simulink model "nl_obsv_hydrotrans_dspace"  (R2021b)
settings: Solver=ode1be  StartTime=0.0  StopTime=inf  FixedStep=ts  MaxStep=ts
PostLoadFcn:
  | if any(exist('dsrtsu_mdlpostloadfcn', 'file') ~= 0), dsrtsu_mdlpostloadfcn('Execute', bdroot); end
InitFcn:
  | , if any(exist('rtifpga_mdlclblib', 'file') ~= 0), rtifpga_mdlclblib('Init', bdroot); end,
  | , if any(exist('dsmpb_private', 'file') ~= 0), dsmpb_private('dsmpb_mdlclblib', 'Init', bdroot); end,
values from neighbouring files (symbols this model uses):
  bd = 5e-2    (= 0.05)    [init_nlobsv_hd.m]
  bf = 0.1    [init_nlobsv_hd.m]
  bm = 0.02    [init_nlobsv_hd.m]
  bp = 0.02    [init_nlobsv_hd.m]
  bulk = 8.36e9    (= 8360000000)    [init_nlobsv_hd.m]
  engine_speed_ref_rpm = 1940    [init_nlobsv_hd.m]
  Jm = 0.05    [init_nlobsv_hd.m]
  Jp = 0.05    [init_nlobsv_hd.m]
  kdrag = 0.01    [init_nlobsv_hd.m]
  kdrag_model = 0.01    [init_nlobsv_hd.m]
  ki_engine = 2.5e-1    (= 0.25)    [init_nlobsv_hd.m]
  kleak = 1e-6    (= 1e-06)    [init_nlobsv_hd.m]
  kp_engine = 2.5e-2    (= 0.025)    [init_nlobsv_hd.m]
  max_domega_m_dt = omega_m_nom_rpm/4    (= 1000)    [init_nlobsv_hd.m]
  ntg = 1    [init_nlobsv_hd.m]
  omega_m_nom_rpm = 4000    [init_nlobsv_hd.m]
  omega_m_ref = 3200    [init_nlobsv_hd.m]
  P0 = eye(4)    [init_nlobsv_hd.m]
  q11 = 10    [init_nlobsv_hd.m]
  q22 = 10    [init_nlobsv_hd.m]
  q33 = 10    [init_nlobsv_hd.m]
  q44 = 2e3    (= 2000)    [init_nlobsv_hd.m]
  ts = 1e-3    (= 0.001)    [init_nlobsv_hd.m]
  tstep = 20    [init_nlobsv_hd.m]
  Vm_nom = 280    [init_nlobsv_hd.m]
  Vp_nom = 210    [init_nlobsv_hd.m]
undefined symbols (not defined in the file or in its folder): consumption, DiscIntNeverNeededParam, rpm_base, rpm_consumption, torque_base, torque_consumption, torque_friction_base
libraries: fl_lib x70, nesl_utility x36, linear_swashplate_ctrl_lib x4, variable_displacement_motor_2_lib x2, variable_displacement_pump_2_lib x2, fixed_displacement_pump_lib x2, relief_valve_lib x2, inverse_shuttle_valve_lib x2, engine_speed_ctrl_kinputs_lib x1, ice_lib x1, gear2_lib x1, flexshaft_lib x1
(part 2 of 2)

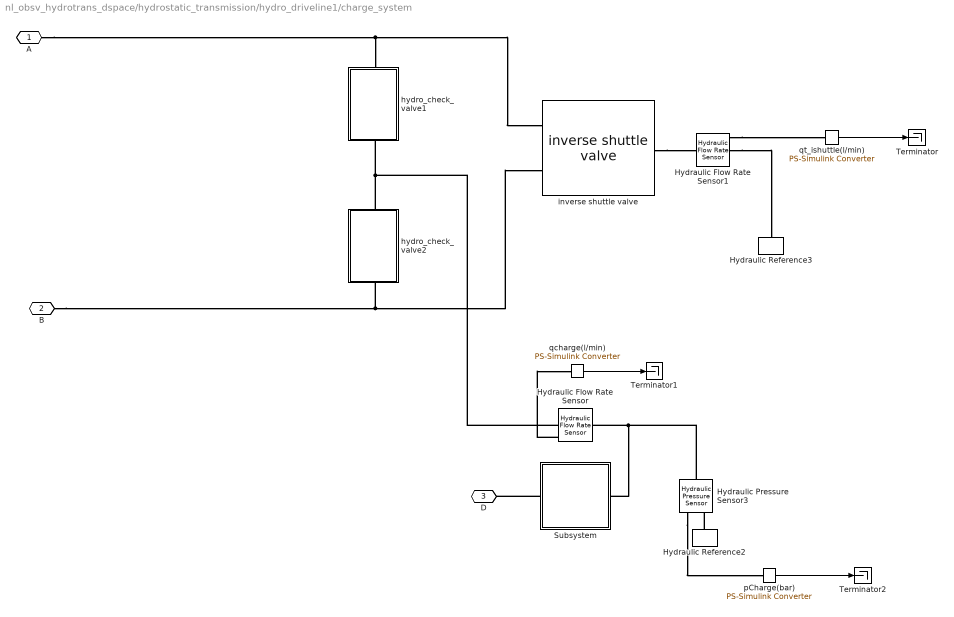
== system nl_obsv_hydrotrans_dspace/hydrostatic_transmission/hydro_driveline1/charge_system ==
  Hydraulic Flow Rate Sensor : fl_lib/Hydraulic/Hydraulic Sensors/Hydraulic Flow Rate Sensor
  Hydraulic Flow Rate Sensor1 : fl_lib/Hydraulic/Hydraulic Sensors/Hydraulic Flow Rate Sensor
  Hydraulic Pressure Sensor3 : fl_lib/Hydraulic/Hydraulic Sensors/Hydraulic Pressure Sensor
  Hydraulic Reference2 : fl_lib/Hydraulic/Hydraulic Elements/Hydraulic Reference
  Hydraulic Reference3 : fl_lib/Hydraulic/Hydraulic Elements/Hydraulic Reference
  Subsystem : Subsystem
  Terminator : Terminator
  Terminator1 : Terminator
  Terminator2 : Terminator
  hydro_check_valve1 : Subsystem
      settings: PortSchema="{\"entries\":[{\"content\":{\"sides\":[{\"content\":{\"connectorIds\":[]},\"type\":\"ConnectorPlacement.EquallySpacedRectSide\",\"uuid\":\"a69fbb91-2279-4dfd-af6f-16497d5f1538\"},{\"content\":{\"connectorIds\":[],\"side\":\"RIGHT\"},\"type\":\"ConnectorPlacement.EquallySpacedRectSide\",\"uuid\":\"52e95d44-b7af-4ccc-8556-a2abd2e724e0\"},{\"content\":{\"connectorIds\":[\"LConn1\"],\"side\":\"TOP\"},\"type\":\"ConnectorPlacement.EquallySpacedRectSide\",\"uuid\":\"2d8c071e-4cd0-4b83-8d45-c175cb858754\"},{\"content\":{\"connectorIds\":[\"RConn1\"],\"side\":\"BOTTOM\"},\"type\":\"ConnectorPlacement.EquallySpacedRectSide\",\"uuid\":\"1baec9dc-757c-4f21-904a-6fc08de72ce1\"}]},\"type\":\"ConnectorPlacement.EquallySpacedConnector\",\"uuid\":\"76990e53-6cb0-4bfe-8c9e-427c41b785f2\"}],\"packageUris\":[\"http://schema.mathworks.com/mf0/Connector/19700101\"],\"version\":\"1.0\"}"
  hydro_check_valve2 : Subsystem
      settings: PortSchema="{\"entries\":[{\"content\":{\"sides\":[{\"content\":{\"connectorIds\":[]},\"type\":\"ConnectorPlacement.EquallySpacedRectSide\",\"uuid\":\"a69fbb91-2279-4dfd-af6f-16497d5f1538\"},{\"content\":{\"connectorIds\":[],\"side\":\"RIGHT\"},\"type\":\"ConnectorPlacement.EquallySpacedRectSide\",\"uuid\":\"52e95d44-b7af-4ccc-8556-a2abd2e724e0\"},{\"content\":{\"connectorIds\":[\"LConn1\"],\"side\":\"TOP\"},\"type\":\"ConnectorPlacement.EquallySpacedRectSide\",\"uuid\":\"2d8c071e-4cd0-4b83-8d45-c175cb858754\"},{\"content\":{\"connectorIds\":[\"RConn1\"],\"side\":\"BOTTOM\"},\"type\":\"ConnectorPlacement.EquallySpacedRectSide\",\"uuid\":\"1baec9dc-757c-4f21-904a-6fc08de72ce1\"}]},\"type\":\"ConnectorPlacement.EquallySpacedConnector\",\"uuid\":\"76990e53-6cb0-4bfe-8c9e-427c41b785f2\"}],\"packageUris\":[\"http://schema.mathworks.com/mf0/Connector/19700101\"],\"version\":\"1.0\"}"
  inverse shuttle valve : inverse_shuttle_valve_lib/inverse shuttle valve  pnom=32 bar  dp_crack=0 bar  dp_reg=0 bar  x_rv_max=2 mm  a0=(2*pi*10)^2 1/s^2  a1=2*2*pi*10 1/s  leak=5e-12 m^3/s/Pa  qA_specify=off  qA_priority=None  qA=0 m^3/s  qA_nominal_specify=off  qA_nominal_unit=m^3/s  qA_nominal_value=1  qB_specify=off  qB_priority=None  qB=0 m^3/s  qB_nominal_specify=off  qB_nominal_unit=m^3/s  qB_nominal_value=1  qP_specify=off  qP_priority=None  qP=0 m^3/s  qP_nominal_specify=off  qP_nominal_unit=m^3/s  qP_nominal_value=1  dp_specify=off  dp_priority=None  dp=0 Pa  dp_nominal_specify=off  dp_nominal_unit=Pa  dp_nominal_value=1  dpAP_specify=off  dpAP_priority=None  dpAP=0 Pa  dpAP_nominal_specify=off  dpAP_nominal_unit=Pa  dpAP_nominal_value=1  dpBP_specify=off  dpBP_priority=None  dpBP=0 Pa  dpBP_nominal_specify=off  dpBP_nominal_unit=Pa  dpBP_nominal_value=1  x_rv_AP_specify=off  x_rv_AP_priority=None  x_rv_AP=0 m  x_rv_AP_nominal_specify=off  x_rv_AP_nominal_unit=m  x_rv_AP_nominal_value=1  x_rv_BP_specify=off  x_rv_BP_priority=None  x_rv_BP=0 m  x_rv_BP_nominal_specify=off  x_rv_BP_nominal_unit=m  x_rv_BP_nominal_value=1  x_rv_AP_flt_specify=off  x_rv_AP_flt_priority=None  x_rv_AP_flt=0 m  x_rv_AP_flt_nominal_specify=off  x_rv_AP_flt_nominal_unit=m  x_rv_AP_flt_nominal_value=1  x_rv_BP_flt_specify=off  x_rv_BP_flt_priority=None  x_rv_BP_flt=0 m  x_rv_BP_flt_nominal_specify=off  x_rv_BP_flt_nominal_unit=m  x_rv_BP_flt_nominal_value=1
      settings: InternalSimscapePortConfiguration="{\"Bottom\":[],\"Left\":[{\"id\":\"cA\",\"label\":\"cA\",\"type\":\"foundation.hydraulic.hydraulic\"},{\"id\":\"cB\",\"label\":\"cB\",\"type\":\"foundation.hydraulic.hydraulic\"}],\"Right\":[{\"id\":\"cP\",\"label\":\"cP\",\"type\":\"foundation.hydraulic.hydraulic\"}],\"Top\":[]}"
  pCharge(bar) : nesl_utility/PS-Simulink Converter  PhysicalDomain=network_engine_domain  SubClassName=ps_output  LeftPortType=input  RightPortType=output  PseudoPeriodic=off  Frequencies=[]  Unit=bar  AffineConversion=on
      settings: SourceProductBaseCode=PW,SS
  qcharge(l/min) : nesl_utility/PS-Simulink Converter  PhysicalDomain=network_engine_domain  SubClassName=ps_output  LeftPortType=input  RightPortType=output  PseudoPeriodic=off  Frequencies=[]  Unit=l/min  AffineConversion=on
      settings: SourceProductBaseCode=PW,SS
  qt_ishuttle(l/min) : nesl_utility/PS-Simulink Converter  PhysicalDomain=network_engine_domain  SubClassName=ps_output  LeftPortType=input  RightPortType=output  PseudoPeriodic=off  Frequencies=[]  Unit=l/min  AffineConversion=on
      settings: SourceProductBaseCode=PW,SS
  A : PMIOPort  Side=Left
  B : PMIOPort  Port=2  Side=Right
  D : PMIOPort  Port=3  Side=Right
  wires:
  qt_ishuttle(l/min)/1 -> Terminator/1
  qcharge(l/min)/1 -> Terminator1/1
  pCharge(bar)/1 -> Terminator2/1
  connections:
  hydro_check_valve2/LConn1 -- Hydraulic Flow Rate Sensor/RConn2 -- hydro_check_valve1/LConn1
  A/RConn1 -- inverse shuttle valve/LConn1 -- hydro_check_valve1/RConn1
  B/RConn1 -- inverse shuttle valve/LConn2 -- hydro_check_valve2/RConn1
  Hydraulic Flow Rate Sensor/RConn1 -- qcharge(l/min)/LConn1
  Hydraulic Pressure Sensor3/LConn1 -- Subsystem/RConn1 -- Hydraulic Flow Rate Sensor/LConn1
  Subsystem/LConn1 -- D/RConn1
  Hydraulic Pressure Sensor3/RConn2 -- pCharge(bar)/LConn1
  Hydraulic Reference2/LConn1 -- Hydraulic Pressure Sensor3/RConn1
  Hydraulic Flow Rate Sensor1/RConn2 -- Hydraulic Reference3/LConn1
  Hydraulic Flow Rate Sensor1/RConn1 -- qt_ishuttle(l/min)/LConn1
  inverse shuttle valve/RConn1 -- Hydraulic Flow Rate Sensor1/LConn1

== system nl_obsv_hydrotrans_dspace/hydrostatic_transmission/hydro_driveline1/vd_ctrl_motor ==
  vd_ref : Inport
  Linear swashplate ctrl2 : linear_swashplate_ctrl_lib/Linear swashplate ctrl  a12=1 1/s  b2=1 1/m/s  k1=100 m  k2=20.5 m  N=5 m  kv=20  xv_specify=off  xv_priority=None  xv=0 m  xv_nominal_specify=off  xv_nominal_unit=m  xv_nominal_value=1  D1_specify=off  D1_priority=None  D1=0  D1_nominal_specify=off  D1_nominal_unit=1  D1_nominal_value=1  D2_specify=off  D2_priority=None  D2=0  D2_nominal_specify=off  D2_nominal_unit=1  D2_nominal_value=1
      settings: InternalSimscapePortConfiguration="{\"Bottom\":[],\"Left\":[{\"id\":\"D_ref\",\"label\":\"Dref\",\"type\":\"input\"}],\"Right\":[{\"id\":\"Dout\",\"label\":\"Dout\",\"type\":\"output\"}],\"Top\":[]}"
  Simulink-PS Converter3 : nesl_utility/Simulink-PS Converter  PhysicalDomain=network_engine_domain  SubClassName=ps_input  LeftPortType=input  RightPortType=output  PseudoPeriodic=off  Frequencies=[]  NoiseDistribution=none  NoiseParameters=[]  Unit=1  AffineConversion=off  FilteringAndDerivatives=provide  SimscapeFilterOrder=1  InputFilterTimeConstant=0.001  UdotUserProvided=0
      settings: SourceProductBaseCode=PW,SS
  vd : PMIOPort  Side=Right
  wires:
  vd_ref/1 -> Simulink-PS Converter3/1
  connections:
  Simulink-PS Converter3/RConn1 -- Linear swashplate ctrl2/LConn1
  Linear swashplate ctrl2/RConn1 -- vd/RConn1

== system nl_obsv_hydrotrans_dspace/hydrostatic_transmission/hydro_driveline1/vd_ctrl_pump ==
  vd_ref : Inport
  Linear swashplate ctrl2 : linear_swashplate_ctrl_lib/Linear swashplate ctrl  a12=1 1/s  b2=1 1/m/s  k1=100 m  k2=20.5 m  N=5 m  kv=20  xv_specify=off  xv_priority=None  xv=0 m  xv_nominal_specify=off  xv_nominal_unit=m  xv_nominal_value=1  D1_specify=off  D1_priority=None  D1=0  D1_nominal_specify=off  D1_nominal_unit=1  D1_nominal_value=1  D2_specify=off  D2_priority=None  D2=0  D2_nominal_specify=off  D2_nominal_unit=1  D2_nominal_value=1
      settings: InternalSimscapePortConfiguration="{\"Bottom\":[],\"Left\":[{\"id\":\"D_ref\",\"label\":\"Dref\",\"type\":\"input\"}],\"Right\":[{\"id\":\"Dout\",\"label\":\"Dout\",\"type\":\"output\"}],\"Top\":[]}"
  Simulink-PS Converter3 : nesl_utility/Simulink-PS Converter  PhysicalDomain=network_engine_domain  SubClassName=ps_input  LeftPortType=input  RightPortType=output  PseudoPeriodic=off  Frequencies=[]  NoiseDistribution=none  NoiseParameters=[]  Unit=1  AffineConversion=off  FilteringAndDerivatives=provide  SimscapeFilterOrder=1  InputFilterTimeConstant=0.001  UdotUserProvided=0
      settings: SourceProductBaseCode=PW,SS
  vd : PMIOPort  Side=Right
  wires:
  vd_ref/1 -> Simulink-PS Converter3/1
  connections:
  Simulink-PS Converter3/RConn1 -- Linear swashplate ctrl2/LConn1
  Linear swashplate ctrl2/RConn1 -- vd/RConn1

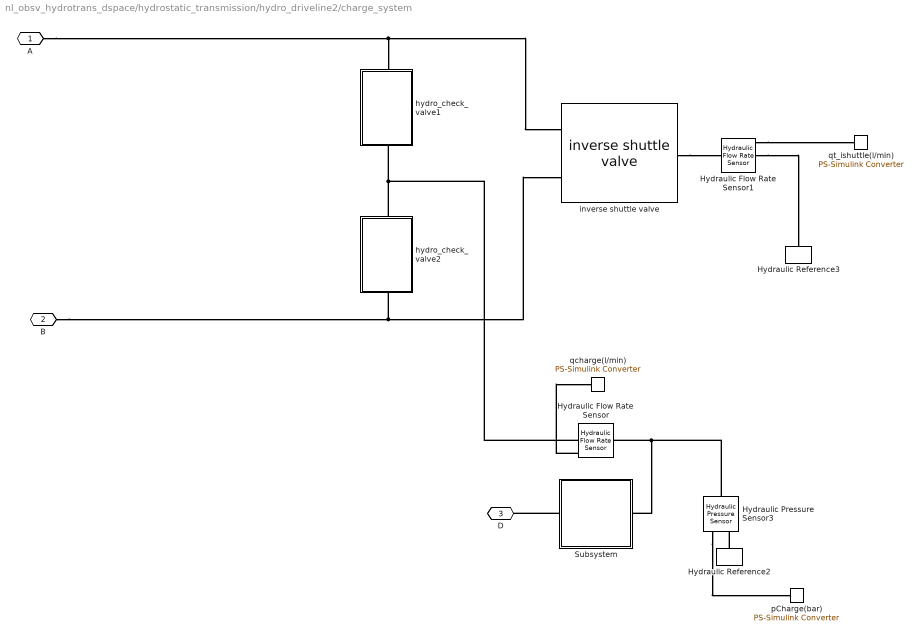
== system nl_obsv_hydrotrans_dspace/hydrostatic_transmission/hydro_driveline2/charge_system ==
  Hydraulic Flow Rate Sensor : fl_lib/Hydraulic/Hydraulic Sensors/Hydraulic Flow Rate Sensor
  Hydraulic Flow Rate Sensor1 : fl_lib/Hydraulic/Hydraulic Sensors/Hydraulic Flow Rate Sensor
  Hydraulic Pressure Sensor3 : fl_lib/Hydraulic/Hydraulic Sensors/Hydraulic Pressure Sensor
  Hydraulic Reference2 : fl_lib/Hydraulic/Hydraulic Elements/Hydraulic Reference
  Hydraulic Reference3 : fl_lib/Hydraulic/Hydraulic Elements/Hydraulic Reference
  Subsystem : Subsystem
  hydro_check_valve1 : Subsystem
      settings: PortSchema="{\"entries\":[{\"content\":{\"sides\":[{\"content\":{\"connectorIds\":[]},\"type\":\"ConnectorPlacement.EquallySpacedRectSide\",\"uuid\":\"a69fbb91-2279-4dfd-af6f-16497d5f1538\"},{\"content\":{\"connectorIds\":[],\"side\":\"RIGHT\"},\"type\":\"ConnectorPlacement.EquallySpacedRectSide\",\"uuid\":\"52e95d44-b7af-4ccc-8556-a2abd2e724e0\"},{\"content\":{\"connectorIds\":[\"LConn1\"],\"side\":\"TOP\"},\"type\":\"ConnectorPlacement.EquallySpacedRectSide\",\"uuid\":\"2d8c071e-4cd0-4b83-8d45-c175cb858754\"},{\"content\":{\"connectorIds\":[\"RConn1\"],\"side\":\"BOTTOM\"},\"type\":\"ConnectorPlacement.EquallySpacedRectSide\",\"uuid\":\"1baec9dc-757c-4f21-904a-6fc08de72ce1\"}]},\"type\":\"ConnectorPlacement.EquallySpacedConnector\",\"uuid\":\"76990e53-6cb0-4bfe-8c9e-427c41b785f2\"}],\"packageUris\":[\"http://schema.mathworks.com/mf0/Connector/19700101\"],\"version\":\"1.0\"}"
  hydro_check_valve2 : Subsystem
      settings: PortSchema="{\"entries\":[{\"content\":{\"sides\":[{\"content\":{\"connectorIds\":[]},\"type\":\"ConnectorPlacement.EquallySpacedRectSide\",\"uuid\":\"a69fbb91-2279-4dfd-af6f-16497d5f1538\"},{\"content\":{\"connectorIds\":[],\"side\":\"RIGHT\"},\"type\":\"ConnectorPlacement.EquallySpacedRectSide\",\"uuid\":\"52e95d44-b7af-4ccc-8556-a2abd2e724e0\"},{\"content\":{\"connectorIds\":[\"LConn1\"],\"side\":\"TOP\"},\"type\":\"ConnectorPlacement.EquallySpacedRectSide\",\"uuid\":\"2d8c071e-4cd0-4b83-8d45-c175cb858754\"},{\"content\":{\"connectorIds\":[\"RConn1\"],\"side\":\"BOTTOM\"},\"type\":\"ConnectorPlacement.EquallySpacedRectSide\",\"uuid\":\"1baec9dc-757c-4f21-904a-6fc08de72ce1\"}]},\"type\":\"ConnectorPlacement.EquallySpacedConnector\",\"uuid\":\"76990e53-6cb0-4bfe-8c9e-427c41b785f2\"}],\"packageUris\":[\"http://schema.mathworks.com/mf0/Connector/19700101\"],\"version\":\"1.0\"}"
  inverse shuttle valve : inverse_shuttle_valve_lib/inverse shuttle valve  pnom=32 bar  dp_crack=0 bar  dp_reg=0 bar  x_rv_max=2 mm  a0=(2*pi*10)^2 1/s^2  a1=2*2*pi*10 1/s  leak=5e-12 m^3/s/Pa  qA_specify=off  qA_priority=None  qA=0 m^3/s  qA_nominal_specify=off  qA_nominal_unit=m^3/s  qA_nominal_value=1  qB_specify=off  qB_priority=None  qB=0 m^3/s  qB_nominal_specify=off  qB_nominal_unit=m^3/s  qB_nominal_value=1  qP_specify=off  qP_priority=None  qP=0 m^3/s  qP_nominal_specify=off  qP_nominal_unit=m^3/s  qP_nominal_value=1  dp_specify=off  dp_priority=None  dp=0 Pa  dp_nominal_specify=off  dp_nominal_unit=Pa  dp_nominal_value=1  dpAP_specify=off  dpAP_priority=None  dpAP=0 Pa  dpAP_nominal_specify=off  dpAP_nominal_unit=Pa  dpAP_nominal_value=1  dpBP_specify=off  dpBP_priority=None  dpBP=0 Pa  dpBP_nominal_specify=off  dpBP_nominal_unit=Pa  dpBP_nominal_value=1  x_rv_AP_specify=off  x_rv_AP_priority=None  x_rv_AP=0 m  x_rv_AP_nominal_specify=off  x_rv_AP_nominal_unit=m  x_rv_AP_nominal_value=1  x_rv_BP_specify=off  x_rv_BP_priority=None  x_rv_BP=0 m  x_rv_BP_nominal_specify=off  x_rv_BP_nominal_unit=m  x_rv_BP_nominal_value=1  x_rv_AP_flt_specify=off  x_rv_AP_flt_priority=None  x_rv_AP_flt=0 m  x_rv_AP_flt_nominal_specify=off  x_rv_AP_flt_nominal_unit=m  x_rv_AP_flt_nominal_value=1  x_rv_BP_flt_specify=off  x_rv_BP_flt_priority=None  x_rv_BP_flt=0 m  x_rv_BP_flt_nominal_specify=off  x_rv_BP_flt_nominal_unit=m  x_rv_BP_flt_nominal_value=1
      settings: InternalSimscapePortConfiguration="{\"Bottom\":[],\"Left\":[{\"id\":\"cA\",\"label\":\"cA\",\"type\":\"foundation.hydraulic.hydraulic\"},{\"id\":\"cB\",\"label\":\"cB\",\"type\":\"foundation.hydraulic.hydraulic\"}],\"Right\":[{\"id\":\"cP\",\"label\":\"cP\",\"type\":\"foundation.hydraulic.hydraulic\"}],\"Top\":[]}"
  pCharge(bar) : nesl_utility/PS-Simulink Converter  PhysicalDomain=network_engine_domain  SubClassName=ps_output  LeftPortType=input  RightPortType=output  PseudoPeriodic=off  Frequencies=[]  Unit=bar  AffineConversion=on
      settings: SourceProductBaseCode=PW,SS
  qcharge(l/min) : nesl_utility/PS-Simulink Converter  PhysicalDomain=network_engine_domain  SubClassName=ps_output  LeftPortType=input  RightPortType=output  PseudoPeriodic=off  Frequencies=[]  Unit=l/min  AffineConversion=on
      settings: SourceProductBaseCode=PW,SS
  qt_ishuttle(l/min) : nesl_utility/PS-Simulink Converter  PhysicalDomain=network_engine_domain  SubClassName=ps_output  LeftPortType=input  RightPortType=output  PseudoPeriodic=off  Frequencies=[]  Unit=l/min  AffineConversion=on
      settings: SourceProductBaseCode=PW,SS
  A : PMIOPort  Side=Left
  B : PMIOPort  Port=2  Side=Right
  D : PMIOPort  Port=3  Side=Right
  connections:
  hydro_check_valve2/LConn1 -- Hydraulic Flow Rate Sensor/RConn2 -- hydro_check_valve1/LConn1
  A/RConn1 -- inverse shuttle valve/LConn1 -- hydro_check_valve1/RConn1
  B/RConn1 -- inverse shuttle valve/LConn2 -- hydro_check_valve2/RConn1
  Hydraulic Flow Rate Sensor/RConn1 -- qcharge(l/min)/LConn1
  Hydraulic Pressure Sensor3/LConn1 -- Subsystem/RConn1 -- Hydraulic Flow Rate Sensor/LConn1
  Subsystem/LConn1 -- D/RConn1
  Hydraulic Pressure Sensor3/RConn2 -- pCharge(bar)/LConn1
  Hydraulic Reference2/LConn1 -- Hydraulic Pressure Sensor3/RConn1
  Hydraulic Flow Rate Sensor1/RConn2 -- Hydraulic Reference3/LConn1
  Hydraulic Flow Rate Sensor1/RConn1 -- qt_ishuttle(l/min)/LConn1
  inverse shuttle valve/RConn1 -- Hydraulic Flow Rate Sensor1/LConn1

== system nl_obsv_hydrotrans_dspace/hydrostatic_transmission/hydro_driveline2/vd_ctrl_motor ==
  vd_ref : Inport
  Linear swashplate ctrl2 : linear_swashplate_ctrl_lib/Linear swashplate ctrl  a12=1 1/s  b2=1 1/m/s  k1=100 m  k2=20.5 m  N=5 m  kv=20  xv_specify=off  xv_priority=None  xv=0 m  xv_nominal_specify=off  xv_nominal_unit=m  xv_nominal_value=1  D1_specify=off  D1_priority=None  D1=0  D1_nominal_specify=off  D1_nominal_unit=1  D1_nominal_value=1  D2_specify=off  D2_priority=None  D2=0  D2_nominal_specify=off  D2_nominal_unit=1  D2_nominal_value=1
      settings: InternalSimscapePortConfiguration="{\"Bottom\":[],\"Left\":[{\"id\":\"D_ref\",\"label\":\"Dref\",\"type\":\"input\"}],\"Right\":[{\"id\":\"Dout\",\"label\":\"Dout\",\"type\":\"output\"}],\"Top\":[]}"
  Simulink-PS Converter3 : nesl_utility/Simulink-PS Converter  PhysicalDomain=network_engine_domain  SubClassName=ps_input  LeftPortType=input  RightPortType=output  PseudoPeriodic=off  Frequencies=[]  NoiseDistribution=none  NoiseParameters=[]  Unit=1  AffineConversion=off  FilteringAndDerivatives=provide  SimscapeFilterOrder=1  InputFilterTimeConstant=0.001  UdotUserProvided=0
      settings: SourceProductBaseCode=PW,SS
  vd : PMIOPort  Side=Right
  wires:
  vd_ref/1 -> Simulink-PS Converter3/1
  connections:
  Linear swashplate ctrl2/RConn1 -- vd/RConn1
  Simulink-PS Converter3/RConn1 -- Linear swashplate ctrl2/LConn1

== system nl_obsv_hydrotrans_dspace/hydrostatic_transmission/hydro_driveline2/vd_ctrl_pump ==
  vd_ref : Inport
  Linear swashplate ctrl2 : linear_swashplate_ctrl_lib/Linear swashplate ctrl  a12=1 1/s  b2=1 1/m/s  k1=100 m  k2=20.5 m  N=5 m  kv=20  xv_specify=off  xv_priority=None  xv=0 m  xv_nominal_specify=off  xv_nominal_unit=m  xv_nominal_value=1  D1_specify=off  D1_priority=None  D1=0  D1_nominal_specify=off  D1_nominal_unit=1  D1_nominal_value=1  D2_specify=off  D2_priority=None  D2=0  D2_nominal_specify=off  D2_nominal_unit=1  D2_nominal_value=1
      settings: InternalSimscapePortConfiguration="{\"Bottom\":[],\"Left\":[{\"id\":\"D_ref\",\"label\":\"Dref\",\"type\":\"input\"}],\"Right\":[{\"id\":\"Dout\",\"label\":\"Dout\",\"type\":\"output\"}],\"Top\":[]}"
  Simulink-PS Converter3 : nesl_utility/Simulink-PS Converter  PhysicalDomain=network_engine_domain  SubClassName=ps_input  LeftPortType=input  RightPortType=output  PseudoPeriodic=off  Frequencies=[]  NoiseDistribution=none  NoiseParameters=[]  Unit=1  AffineConversion=off  FilteringAndDerivatives=provide  SimscapeFilterOrder=1  InputFilterTimeConstant=0.001  UdotUserProvided=0
      settings: SourceProductBaseCode=PW,SS
  vd : PMIOPort  Side=Right
  wires:
  vd_ref/1 -> Simulink-PS Converter3/1
  connections:
  Linear swashplate ctrl2/RConn1 -- vd/RConn1
  Simulink-PS Converter3/RConn1 -- Linear swashplate ctrl2/LConn1

== system nl_obsv_hydrotrans_dspace/hydrostatic_transmission/hydro_driveline1/charge_system/Subsystem ==
  Fixed displacement pump : fixed_displacement_pump_lib/Fixed displacement pump  max_Dv=27 cm^3/rev  inertia_pump=0.05 kg*m^2  oil_vol=2.0 l  bp=0.0025 N*m/(rad/s)  lk=1e-6 m  t_specify=off  t_priority=None  t=0 N*m  t_nominal_specify=off  t_nominal_unit=N*m  t_nominal_value=1  q_specify=off  q_priority=None  q=0 m^3/s  q_nominal_specify=off  q_nominal_unit=m^3/s  q_nominal_value=1  qt_specify=off  qt_priority=None  qt=0 m^3/s  qt_nominal_specify=off  qt_nominal_unit=m^3/s  qt_nominal_value=1  qleak_specify=off  qleak_priority=None  qleak=0 m^3/s  qleak_nominal_specify=off  qleak_nominal_unit=m^3/s  qleak_nominal_value=1  Dv_specify=off  Dv_priority=None  Dv=0 cm^3  Dv_nominal_specify=off  Dv_nominal_unit=cm^3  Dv_nominal_value=1  dp_specify=off  dp_priority=None  dp=0 Pa  dp_nominal_specify=off  dp_nominal_unit=Pa  dp_nominal_value=1  we_specify=off  we_priority=None  we=0 rad/s  we_nominal_specify=off  we_nominal_unit=rad/s  we_nominal_value=1
      settings: InternalSimscapePortConfiguration="{\"Bottom\":[],\"Left\":[{\"id\":\"C\",\"label\":\"C\",\"type\":\"foundation.mechanical.rotational.rotational\"}],\"Right\":[{\"id\":\"A\",\"label\":\"A\",\"type\":\"foundation.hydraulic.hydraulic\"},{\"id\":\"B\",\"label\":\"B\",\"type\":\"foundation.hydraulic.hydraulic\"}],\"Top\":[]}"
  Hydraulic Reference3 : fl_lib/Hydraulic/Hydraulic Elements/Hydraulic Reference
  Hydraulic Reference4 : fl_lib/Hydraulic/Hydraulic Elements/Hydraulic Reference
  relief valve : relief_valve_lib/relief valve  dp_ref=32 bar  pnom=32 bar  p_set=32 bar  p_reg=12 bar  x_rv_max=12.0 mm  qA_specify=off  qA_priority=None  qA=0 m^3/s  qA_nominal_specify=off  qA_nominal_unit=m^3/s  qA_nominal_value=1  qB_specify=off  qB_priority=None  qB=0 m^3/s  qB_nominal_specify=off  qB_nominal_unit=m^3/s  qB_nominal_value=1  dp_specify=off  dp_priority=None  dp=0 Pa  dp_nominal_specify=off  dp_nominal_unit=Pa  dp_nominal_value=1  x_rv_specify=off  x_rv_priority=None  x_rv=0 m  x_rv_nominal_specify=off  x_rv_nominal_unit=m  x_rv_nominal_value=1  x_rv_flt_specify=off  x_rv_flt_priority=None  x_rv_flt=0 m  x_rv_flt_nominal_specify=off  x_rv_flt_nominal_unit=m  x_rv_flt_nominal_value=1
      settings: LogSimulationData=on  InternalSimscapePortConfiguration="{\"Bottom\":[],\"Left\":[{\"id\":\"cA\",\"label\":\"cA\",\"type\":\"foundation.hydraulic.hydraulic\"}],\"Right\":[{\"id\":\"cB\",\"label\":\"cB\",\"type\":\"foundation.hydraulic.hydraulic\"}],\"Top\":[]}"
  ps : PMIOPort  Side=Right
  D : PMIOPort  Port=2  Side=Left
  connections:
  Fixed displacement pump/RConn1 -- ps/RConn1 -- relief valve/LConn1
  Hydraulic Reference4/LConn1 -- relief valve/RConn1
  Fixed displacement pump/RConn2 -- Hydraulic Reference3/LConn1
  Fixed displacement pump/LConn1 -- D/RConn1

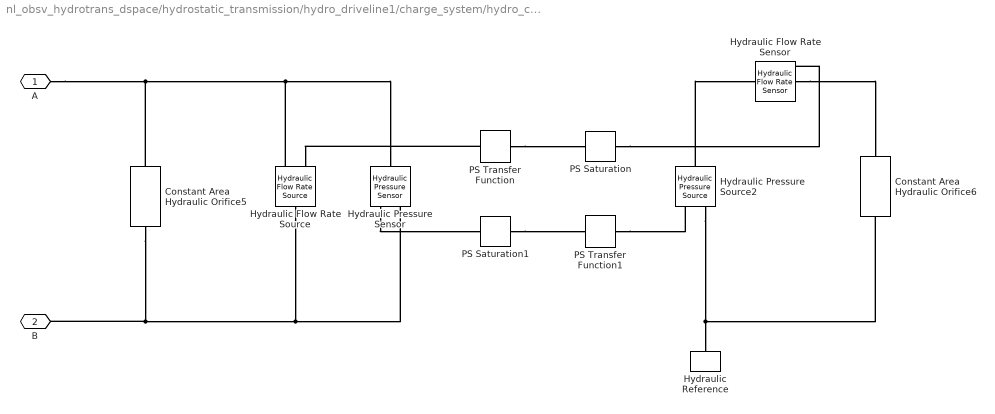
== system nl_obsv_hydrotrans_dspace/hydrostatic_transmission/hydro_driveline1/charge_system/hydro_check_valve1 ==
  Constant Area Hydraulic Orifice5 : fl_lib/Hydraulic/Hydraulic Elements/Constant Area Hydraulic Orifice  area=1e-4 mm^2  C_d=1  lam_spec=1  B_lam=0.999  Re_cr=12  q_specify=off  q_priority=None  q=0.001 m^3/s  q_nominal_specify=off  q_nominal_unit=m^3/s  q_nominal_value=1  p_specify=off  p_priority=None  p=0 Pa  p_nominal_specify=off  p_nominal_unit=Pa  p_nominal_value=1
      settings: SourceProductBaseCode=SS  InternalSimscapePortConfiguration="{\"Bottom\":[],\"Left\":[{\"id\":\"A\",\"label\":\"A\",\"type\":\"foundation.hydraulic.hydraulic\"}],\"Right\":[{\"id\":\"B\",\"label\":\"B\",\"type\":\"foundation.hydraulic.hydraulic\"}],\"Top\":[]}"
  Constant Area Hydraulic Orifice6 : fl_lib/Hydraulic/Hydraulic Elements/Constant Area Hydraulic Orifice  area=4 mm^2  C_d=1  lam_spec=1  B_lam=0.999  Re_cr=12  q_specify=off  q_priority=None  q=0.001 m^3/s  q_nominal_specify=off  q_nominal_unit=m^3/s  q_nominal_value=1  p_specify=off  p_priority=None  p=0 Pa  p_nominal_specify=off  p_nominal_unit=Pa  p_nominal_value=1
      settings: SourceProductBaseCode=SS  InternalSimscapePortConfiguration="{\"Bottom\":[],\"Left\":[{\"id\":\"A\",\"label\":\"A\",\"type\":\"foundation.hydraulic.hydraulic\"}],\"Right\":[{\"id\":\"B\",\"label\":\"B\",\"type\":\"foundation.hydraulic.hydraulic\"}],\"Top\":[]}"
  Hydraulic Flow Rate Sensor : fl_lib/Hydraulic/Hydraulic Sensors/Hydraulic Flow Rate Sensor
  Hydraulic Flow Rate Source : fl_lib/Hydraulic/Hydraulic Sources/Hydraulic Flow Rate Source
      settings: SourceProductBaseCode=SS  InternalSimscapePortConfiguration="{\"Bottom\":[],\"Left\":[{\"id\":\"P\",\"label\":\"P\",\"type\":\"foundation.hydraulic.hydraulic\"}],\"Right\":[{\"id\":\"S\",\"label\":\"S\",\"type\":\"input\"},{\"id\":\"T\",\"label\":\"T\",\"type\":\"foundation.hydraulic.hydraulic\"}],\"Top\":[]}"
  Hydraulic Pressure Sensor : fl_lib/Hydraulic/Hydraulic Sensors/Hydraulic Pressure Sensor
  Hydraulic Pressure Source2 : fl_lib/Hydraulic/Hydraulic Sources/Hydraulic Pressure Source
      settings: SourceProductBaseCode=SS  InternalSimscapePortConfiguration="{\"Bottom\":[],\"Left\":[{\"id\":\"P\",\"label\":\"P\",\"type\":\"foundation.hydraulic.hydraulic\"}],\"Right\":[{\"id\":\"S\",\"label\":\"S\",\"type\":\"input\"},{\"id\":\"T\",\"label\":\"T\",\"type\":\"foundation.hydraulic.hydraulic\"}],\"Top\":[]}"
  Hydraulic Reference : fl_lib/Hydraulic/Hydraulic Elements/Hydraulic Reference
  PS Saturation : fl_lib/Physical Signals/Nonlinear Operators/PS Saturation  upper_limit=inf m^3/s  lower_limit=0 m^3/s
      settings: SourceProductBaseCode=SS
  PS Saturation1 : fl_lib/Physical Signals/Nonlinear Operators/PS Saturation  upper_limit=inf Pa  lower_limit=0 Pa
      settings: SourceProductBaseCode=SS
  PS Transfer Function : fl_lib/Physical Signals/Linear Operators/PS Transfer Function  transfer_function_type=foundation.enum.transfer_function_type.lag  T=ts s  T1=2 s  T2=1 s  y0=0 m^3/s
      settings: SourceProductBaseCode=SS  InternalSimscapePortConfiguration="{\"Bottom\":[],\"Left\":[{\"id\":\"U\",\"label\":\"\",\"type\":\"input\"}],\"Right\":[{\"id\":\"Y\",\"label\":\"\",\"type\":\"output\"}],\"Top\":[]}"
  PS Transfer Function1 : fl_lib/Physical Signals/Linear Operators/PS Transfer Function  transfer_function_type=foundation.enum.transfer_function_type.lag  T=ts s  T1=2 s  T2=1 s  y0=0 Pa
      settings: SourceProductBaseCode=SS  InternalSimscapePortConfiguration="{\"Bottom\":[],\"Left\":[{\"id\":\"U\",\"label\":\"\",\"type\":\"input\"}],\"Right\":[{\"id\":\"Y\",\"label\":\"\",\"type\":\"output\"}],\"Top\":[]}"
  A : PMIOPort  Side=Left
  B : PMIOPort  Port=2  Side=Right
  connections:
  Hydraulic Flow Rate Sensor/RConn2 -- Constant Area Hydraulic Orifice6/LConn1
  Constant Area Hydraulic Orifice6/RConn1 -- Hydraulic Reference/LConn1 -- Hydraulic Pressure Source2/RConn2
  Hydraulic Pressure Source2/LConn1 -- Hydraulic Flow Rate Sensor/LConn1
  Hydraulic Flow Rate Source/LConn1 -- Hydraulic Pressure Sensor/RConn1 -- Constant Area Hydraulic Orifice5/RConn1 -- B/RConn1
  PS Saturation/LConn1 -- Hydraulic Flow Rate Sensor/RConn1
  PS Transfer Function1/RConn1 -- Hydraulic Pressure Source2/RConn1
  Hydraulic Pressure Sensor/RConn2 -- PS Saturation1/LConn1
  Hydraulic Flow Rate Source/RConn2 -- Hydraulic Pressure Sensor/LConn1 -- A/RConn1 -- Constant Area Hydraulic Orifice5/LConn1
  PS Transfer Function/RConn1 -- Hydraulic Flow Rate Source/RConn1
  PS Saturation1/RConn1 -- PS Transfer Function1/LConn1
  PS Transfer Function/LConn1 -- PS Saturation/RConn1

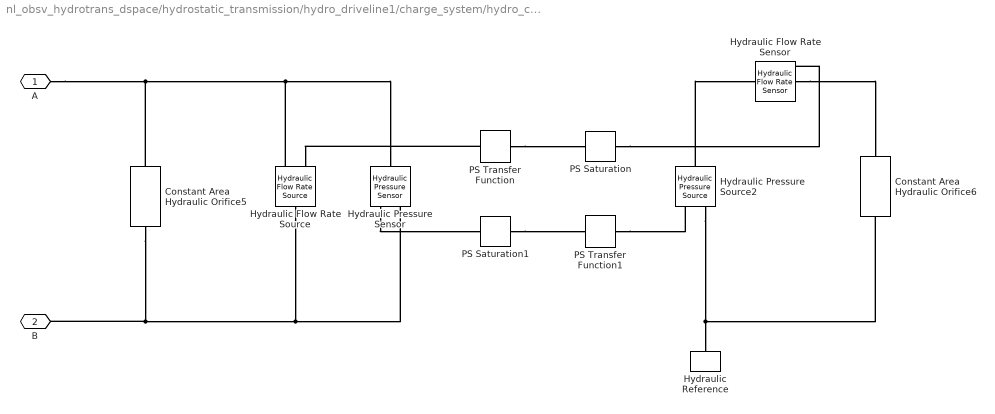
== system nl_obsv_hydrotrans_dspace/hydrostatic_transmission/hydro_driveline1/charge_system/hydro_check_valve2 ==
  Constant Area Hydraulic Orifice5 : fl_lib/Hydraulic/Hydraulic Elements/Constant Area Hydraulic Orifice  area=1e-4 mm^2  C_d=1  lam_spec=1  B_lam=0.999  Re_cr=12  q_specify=off  q_priority=None  q=0.001 m^3/s  q_nominal_specify=off  q_nominal_unit=m^3/s  q_nominal_value=1  p_specify=off  p_priority=None  p=0 Pa  p_nominal_specify=off  p_nominal_unit=Pa  p_nominal_value=1
      settings: SourceProductBaseCode=SS  InternalSimscapePortConfiguration="{\"Bottom\":[],\"Left\":[{\"id\":\"A\",\"label\":\"A\",\"type\":\"foundation.hydraulic.hydraulic\"}],\"Right\":[{\"id\":\"B\",\"label\":\"B\",\"type\":\"foundation.hydraulic.hydraulic\"}],\"Top\":[]}"
  Constant Area Hydraulic Orifice6 : fl_lib/Hydraulic/Hydraulic Elements/Constant Area Hydraulic Orifice  area=4 mm^2  C_d=1  lam_spec=1  B_lam=0.999  Re_cr=12  q_specify=off  q_priority=None  q=0.001 m^3/s  q_nominal_specify=off  q_nominal_unit=m^3/s  q_nominal_value=1  p_specify=off  p_priority=None  p=0 Pa  p_nominal_specify=off  p_nominal_unit=Pa  p_nominal_value=1
      settings: SourceProductBaseCode=SS  InternalSimscapePortConfiguration="{\"Bottom\":[],\"Left\":[{\"id\":\"A\",\"label\":\"A\",\"type\":\"foundation.hydraulic.hydraulic\"}],\"Right\":[{\"id\":\"B\",\"label\":\"B\",\"type\":\"foundation.hydraulic.hydraulic\"}],\"Top\":[]}"
  Hydraulic Flow Rate Sensor : fl_lib/Hydraulic/Hydraulic Sensors/Hydraulic Flow Rate Sensor
  Hydraulic Flow Rate Source : fl_lib/Hydraulic/Hydraulic Sources/Hydraulic Flow Rate Source
      settings: SourceProductBaseCode=SS  InternalSimscapePortConfiguration="{\"Bottom\":[],\"Left\":[{\"id\":\"P\",\"label\":\"P\",\"type\":\"foundation.hydraulic.hydraulic\"}],\"Right\":[{\"id\":\"S\",\"label\":\"S\",\"type\":\"input\"},{\"id\":\"T\",\"label\":\"T\",\"type\":\"foundation.hydraulic.hydraulic\"}],\"Top\":[]}"
  Hydraulic Pressure Sensor : fl_lib/Hydraulic/Hydraulic Sensors/Hydraulic Pressure Sensor
  Hydraulic Pressure Source2 : fl_lib/Hydraulic/Hydraulic Sources/Hydraulic Pressure Source
      settings: SourceProductBaseCode=SS  InternalSimscapePortConfiguration="{\"Bottom\":[],\"Left\":[{\"id\":\"P\",\"label\":\"P\",\"type\":\"foundation.hydraulic.hydraulic\"}],\"Right\":[{\"id\":\"S\",\"label\":\"S\",\"type\":\"input\"},{\"id\":\"T\",\"label\":\"T\",\"type\":\"foundation.hydraulic.hydraulic\"}],\"Top\":[]}"
  Hydraulic Reference : fl_lib/Hydraulic/Hydraulic Elements/Hydraulic Reference
  PS Saturation : fl_lib/Physical Signals/Nonlinear Operators/PS Saturation  upper_limit=inf m^3/s  lower_limit=0 m^3/s
      settings: SourceProductBaseCode=SS
  PS Saturation1 : fl_lib/Physical Signals/Nonlinear Operators/PS Saturation  upper_limit=inf Pa  lower_limit=0 Pa
      settings: SourceProductBaseCode=SS
  PS Transfer Function : fl_lib/Physical Signals/Linear Operators/PS Transfer Function  transfer_function_type=foundation.enum.transfer_function_type.lag  T=ts s  T1=2 s  T2=1 s  y0=0 m^3/s
      settings: SourceProductBaseCode=SS  InternalSimscapePortConfiguration="{\"Bottom\":[],\"Left\":[{\"id\":\"U\",\"label\":\"\",\"type\":\"input\"}],\"Right\":[{\"id\":\"Y\",\"label\":\"\",\"type\":\"output\"}],\"Top\":[]}"
  PS Transfer Function1 : fl_lib/Physical Signals/Linear Operators/PS Transfer Function  transfer_function_type=foundation.enum.transfer_function_type.lag  T=ts s  T1=2 s  T2=1 s  y0=0 Pa
      settings: SourceProductBaseCode=SS  InternalSimscapePortConfiguration="{\"Bottom\":[],\"Left\":[{\"id\":\"U\",\"label\":\"\",\"type\":\"input\"}],\"Right\":[{\"id\":\"Y\",\"label\":\"\",\"type\":\"output\"}],\"Top\":[]}"
  A : PMIOPort  Side=Left
  B : PMIOPort  Port=2  Side=Right
  connections:
  PS Transfer Function/LConn1 -- PS Saturation/RConn1
  PS Saturation1/RConn1 -- PS Transfer Function1/LConn1
  PS Transfer Function/RConn1 -- Hydraulic Flow Rate Source/RConn1
  Constant Area Hydraulic Orifice5/LConn1 -- A/RConn1 -- Hydraulic Pressure Sensor/LConn1 -- Hydraulic Flow Rate Source/RConn2
  Hydraulic Pressure Sensor/RConn2 -- PS Saturation1/LConn1
  PS Transfer Function1/RConn1 -- Hydraulic Pressure Source2/RConn1
  PS Saturation/LConn1 -- Hydraulic Flow Rate Sensor/RConn1
  B/RConn1 -- Constant Area Hydraulic Orifice5/RConn1 -- Hydraulic Pressure Sensor/RConn1 -- Hydraulic Flow Rate Source/LConn1
  Hydraulic Pressure Source2/LConn1 -- Hydraulic Flow Rate Sensor/LConn1
  Hydraulic Pressure Source2/RConn2 -- Hydraulic Reference/LConn1 -- Constant Area Hydraulic Orifice6/RConn1
  Hydraulic Flow Rate Sensor/RConn2 -- Constant Area Hydraulic Orifice6/LConn1

== system nl_obsv_hydrotrans_dspace/hydrostatic_transmission/hydro_driveline2/charge_system/Subsystem ==
  Fixed displacement pump : fixed_displacement_pump_lib/Fixed displacement pump  max_Dv=27 cm^3/rev  inertia_pump=0.05 kg*m^2  oil_vol=2.0 l  bp=0.0025 N*m/(rad/s)  lk=1e-6 m  t_specify=off  t_priority=None  t=0 N*m  t_nominal_specify=off  t_nominal_unit=N*m  t_nominal_value=1  q_specify=off  q_priority=None  q=0 m^3/s  q_nominal_specify=off  q_nominal_unit=m^3/s  q_nominal_value=1  qt_specify=off  qt_priority=None  qt=0 m^3/s  qt_nominal_specify=off  qt_nominal_unit=m^3/s  qt_nominal_value=1  qleak_specify=off  qleak_priority=None  qleak=0 m^3/s  qleak_nominal_specify=off  qleak_nominal_unit=m^3/s  qleak_nominal_value=1  Dv_specify=off  Dv_priority=None  Dv=0 cm^3  Dv_nominal_specify=off  Dv_nominal_unit=cm^3  Dv_nominal_value=1  dp_specify=off  dp_priority=None  dp=0 Pa  dp_nominal_specify=off  dp_nominal_unit=Pa  dp_nominal_value=1  we_specify=off  we_priority=None  we=0 rad/s  we_nominal_specify=off  we_nominal_unit=rad/s  we_nominal_value=1
      settings: InternalSimscapePortConfiguration="{\"Bottom\":[],\"Left\":[{\"id\":\"C\",\"label\":\"C\",\"type\":\"foundation.mechanical.rotational.rotational\"}],\"Right\":[{\"id\":\"A\",\"label\":\"A\",\"type\":\"foundation.hydraulic.hydraulic\"},{\"id\":\"B\",\"label\":\"B\",\"type\":\"foundation.hydraulic.hydraulic\"}],\"Top\":[]}"
  Hydraulic Reference3 : fl_lib/Hydraulic/Hydraulic Elements/Hydraulic Reference
  Hydraulic Reference4 : fl_lib/Hydraulic/Hydraulic Elements/Hydraulic Reference
  relief valve : relief_valve_lib/relief valve  dp_ref=32 bar  pnom=32 bar  p_set=32 bar  p_reg=12 bar  x_rv_max=12.0 mm  qA_specify=off  qA_priority=None  qA=0 m^3/s  qA_nominal_specify=off  qA_nominal_unit=m^3/s  qA_nominal_value=1  qB_specify=off  qB_priority=None  qB=0 m^3/s  qB_nominal_specify=off  qB_nominal_unit=m^3/s  qB_nominal_value=1  dp_specify=off  dp_priority=None  dp=0 Pa  dp_nominal_specify=off  dp_nominal_unit=Pa  dp_nominal_value=1  x_rv_specify=off  x_rv_priority=None  x_rv=0 m  x_rv_nominal_specify=off  x_rv_nominal_unit=m  x_rv_nominal_value=1  x_rv_flt_specify=off  x_rv_flt_priority=None  x_rv_flt=0 m  x_rv_flt_nominal_specify=off  x_rv_flt_nominal_unit=m  x_rv_flt_nominal_value=1
      settings: LogSimulationData=on  InternalSimscapePortConfiguration="{\"Bottom\":[],\"Left\":[{\"id\":\"cA\",\"label\":\"cA\",\"type\":\"foundation.hydraulic.hydraulic\"}],\"Right\":[{\"id\":\"cB\",\"label\":\"cB\",\"type\":\"foundation.hydraulic.hydraulic\"}],\"Top\":[]}"
  ps : PMIOPort  Side=Right
  D : PMIOPort  Port=2  Side=Left
  connections:
  Fixed displacement pump/RConn1 -- ps/RConn1 -- relief valve/LConn1
  Hydraulic Reference4/LConn1 -- relief valve/RConn1
  Fixed displacement pump/RConn2 -- Hydraulic Reference3/LConn1
  Fixed displacement pump/LConn1 -- D/RConn1

== system nl_obsv_hydrotrans_dspace/hydrostatic_transmission/hydro_driveline2/charge_system/hydro_check_valve1 ==
  Constant Area Hydraulic Orifice5 : fl_lib/Hydraulic/Hydraulic Elements/Constant Area Hydraulic Orifice  area=1e-4 mm^2  C_d=1  lam_spec=1  B_lam=0.999  Re_cr=12  q_specify=off  q_priority=None  q=0.001 m^3/s  q_nominal_specify=off  q_nominal_unit=m^3/s  q_nominal_value=1  p_specify=off  p_priority=None  p=0 Pa  p_nominal_specify=off  p_nominal_unit=Pa  p_nominal_value=1
      settings: SourceProductBaseCode=SS  InternalSimscapePortConfiguration="{\"Bottom\":[],\"Left\":[{\"id\":\"A\",\"label\":\"A\",\"type\":\"foundation.hydraulic.hydraulic\"}],\"Right\":[{\"id\":\"B\",\"label\":\"B\",\"type\":\"foundation.hydraulic.hydraulic\"}],\"Top\":[]}"
  Constant Area Hydraulic Orifice6 : fl_lib/Hydraulic/Hydraulic Elements/Constant Area Hydraulic Orifice  area=4 mm^2  C_d=1  lam_spec=1  B_lam=0.999  Re_cr=12  q_specify=off  q_priority=None  q=0.001 m^3/s  q_nominal_specify=off  q_nominal_unit=m^3/s  q_nominal_value=1  p_specify=off  p_priority=None  p=0 Pa  p_nominal_specify=off  p_nominal_unit=Pa  p_nominal_value=1
      settings: SourceProductBaseCode=SS  InternalSimscapePortConfiguration="{\"Bottom\":[],\"Left\":[{\"id\":\"A\",\"label\":\"A\",\"type\":\"foundation.hydraulic.hydraulic\"}],\"Right\":[{\"id\":\"B\",\"label\":\"B\",\"type\":\"foundation.hydraulic.hydraulic\"}],\"Top\":[]}"
  Hydraulic Flow Rate Sensor : fl_lib/Hydraulic/Hydraulic Sensors/Hydraulic Flow Rate Sensor
  Hydraulic Flow Rate Source : fl_lib/Hydraulic/Hydraulic Sources/Hydraulic Flow Rate Source
      settings: SourceProductBaseCode=SS  InternalSimscapePortConfiguration="{\"Bottom\":[],\"Left\":[{\"id\":\"P\",\"label\":\"P\",\"type\":\"foundation.hydraulic.hydraulic\"}],\"Right\":[{\"id\":\"S\",\"label\":\"S\",\"type\":\"input\"},{\"id\":\"T\",\"label\":\"T\",\"type\":\"foundation.hydraulic.hydraulic\"}],\"Top\":[]}"
  Hydraulic Pressure Sensor : fl_lib/Hydraulic/Hydraulic Sensors/Hydraulic Pressure Sensor
  Hydraulic Pressure Source2 : fl_lib/Hydraulic/Hydraulic Sources/Hydraulic Pressure Source
      settings: SourceProductBaseCode=SS  InternalSimscapePortConfiguration="{\"Bottom\":[],\"Left\":[{\"id\":\"P\",\"label\":\"P\",\"type\":\"foundation.hydraulic.hydraulic\"}],\"Right\":[{\"id\":\"S\",\"label\":\"S\",\"type\":\"input\"},{\"id\":\"T\",\"label\":\"T\",\"type\":\"foundation.hydraulic.hydraulic\"}],\"Top\":[]}"
  Hydraulic Reference : fl_lib/Hydraulic/Hydraulic Elements/Hydraulic Reference
  PS Saturation : fl_lib/Physical Signals/Nonlinear Operators/PS Saturation  upper_limit=inf m^3/s  lower_limit=0 m^3/s
      settings: SourceProductBaseCode=SS
  PS Saturation1 : fl_lib/Physical Signals/Nonlinear Operators/PS Saturation  upper_limit=inf Pa  lower_limit=0 Pa
      settings: SourceProductBaseCode=SS
  PS Transfer Function : fl_lib/Physical Signals/Linear Operators/PS Transfer Function  transfer_function_type=foundation.enum.transfer_function_type.lag  T=ts s  T1=2 s  T2=1 s  y0=0 m^3/s
      settings: SourceProductBaseCode=SS  InternalSimscapePortConfiguration="{\"Bottom\":[],\"Left\":[{\"id\":\"U\",\"label\":\"\",\"type\":\"input\"}],\"Right\":[{\"id\":\"Y\",\"label\":\"\",\"type\":\"output\"}],\"Top\":[]}"
  PS Transfer Function1 : fl_lib/Physical Signals/Linear Operators/PS Transfer Function  transfer_function_type=foundation.enum.transfer_function_type.lag  T=ts s  T1=2 s  T2=1 s  y0=0 Pa
      settings: SourceProductBaseCode=SS  InternalSimscapePortConfiguration="{\"Bottom\":[],\"Left\":[{\"id\":\"U\",\"label\":\"\",\"type\":\"input\"}],\"Right\":[{\"id\":\"Y\",\"label\":\"\",\"type\":\"output\"}],\"Top\":[]}"
  A : PMIOPort  Side=Left
  B : PMIOPort  Port=2  Side=Right
  connections:
  Hydraulic Flow Rate Sensor/RConn2 -- Constant Area Hydraulic Orifice6/LConn1
  Constant Area Hydraulic Orifice6/RConn1 -- Hydraulic Reference/LConn1 -- Hydraulic Pressure Source2/RConn2
  Hydraulic Pressure Source2/LConn1 -- Hydraulic Flow Rate Sensor/LConn1
  Hydraulic Flow Rate Source/LConn1 -- Hydraulic Pressure Sensor/RConn1 -- Constant Area Hydraulic Orifice5/RConn1 -- B/RConn1
  PS Saturation/LConn1 -- Hydraulic Flow Rate Sensor/RConn1
  PS Transfer Function1/RConn1 -- Hydraulic Pressure Source2/RConn1
  Hydraulic Pressure Sensor/RConn2 -- PS Saturation1/LConn1
  Hydraulic Flow Rate Source/RConn2 -- Hydraulic Pressure Sensor/LConn1 -- A/RConn1 -- Constant Area Hydraulic Orifice5/LConn1
  PS Transfer Function/RConn1 -- Hydraulic Flow Rate Source/RConn1
  PS Saturation1/RConn1 -- PS Transfer Function1/LConn1
  PS Transfer Function/LConn1 -- PS Saturation/RConn1

== system nl_obsv_hydrotrans_dspace/hydrostatic_transmission/hydro_driveline2/charge_system/hydro_check_valve2 ==
  Constant Area Hydraulic Orifice5 : fl_lib/Hydraulic/Hydraulic Elements/Constant Area Hydraulic Orifice  area=1e-4 mm^2  C_d=1  lam_spec=1  B_lam=0.999  Re_cr=12  q_specify=off  q_priority=None  q=0.001 m^3/s  q_nominal_specify=off  q_nominal_unit=m^3/s  q_nominal_value=1  p_specify=off  p_priority=None  p=0 Pa  p_nominal_specify=off  p_nominal_unit=Pa  p_nominal_value=1
      settings: SourceProductBaseCode=SS  InternalSimscapePortConfiguration="{\"Bottom\":[],\"Left\":[{\"id\":\"A\",\"label\":\"A\",\"type\":\"foundation.hydraulic.hydraulic\"}],\"Right\":[{\"id\":\"B\",\"label\":\"B\",\"type\":\"foundation.hydraulic.hydraulic\"}],\"Top\":[]}"
  Constant Area Hydraulic Orifice6 : fl_lib/Hydraulic/Hydraulic Elements/Constant Area Hydraulic Orifice  area=4 mm^2  C_d=1  lam_spec=1  B_lam=0.999  Re_cr=12  q_specify=off  q_priority=None  q=0.001 m^3/s  q_nominal_specify=off  q_nominal_unit=m^3/s  q_nominal_value=1  p_specify=off  p_priority=None  p=0 Pa  p_nominal_specify=off  p_nominal_unit=Pa  p_nominal_value=1
      settings: SourceProductBaseCode=SS  InternalSimscapePortConfiguration="{\"Bottom\":[],\"Left\":[{\"id\":\"A\",\"label\":\"A\",\"type\":\"foundation.hydraulic.hydraulic\"}],\"Right\":[{\"id\":\"B\",\"label\":\"B\",\"type\":\"foundation.hydraulic.hydraulic\"}],\"Top\":[]}"
  Hydraulic Flow Rate Sensor : fl_lib/Hydraulic/Hydraulic Sensors/Hydraulic Flow Rate Sensor
  Hydraulic Flow Rate Source : fl_lib/Hydraulic/Hydraulic Sources/Hydraulic Flow Rate Source
      settings: SourceProductBaseCode=SS  InternalSimscapePortConfiguration="{\"Bottom\":[],\"Left\":[{\"id\":\"P\",\"label\":\"P\",\"type\":\"foundation.hydraulic.hydraulic\"}],\"Right\":[{\"id\":\"S\",\"label\":\"S\",\"type\":\"input\"},{\"id\":\"T\",\"label\":\"T\",\"type\":\"foundation.hydraulic.hydraulic\"}],\"Top\":[]}"
  Hydraulic Pressure Sensor : fl_lib/Hydraulic/Hydraulic Sensors/Hydraulic Pressure Sensor
  Hydraulic Pressure Source2 : fl_lib/Hydraulic/Hydraulic Sources/Hydraulic Pressure Source
      settings: SourceProductBaseCode=SS  InternalSimscapePortConfiguration="{\"Bottom\":[],\"Left\":[{\"id\":\"P\",\"label\":\"P\",\"type\":\"foundation.hydraulic.hydraulic\"}],\"Right\":[{\"id\":\"S\",\"label\":\"S\",\"type\":\"input\"},{\"id\":\"T\",\"label\":\"T\",\"type\":\"foundation.hydraulic.hydraulic\"}],\"Top\":[]}"
  Hydraulic Reference : fl_lib/Hydraulic/Hydraulic Elements/Hydraulic Reference
  PS Saturation : fl_lib/Physical Signals/Nonlinear Operators/PS Saturation  upper_limit=inf m^3/s  lower_limit=0 m^3/s
      settings: SourceProductBaseCode=SS
  PS Saturation1 : fl_lib/Physical Signals/Nonlinear Operators/PS Saturation  upper_limit=inf Pa  lower_limit=0 Pa
      settings: SourceProductBaseCode=SS
  PS Transfer Function : fl_lib/Physical Signals/Linear Operators/PS Transfer Function  transfer_function_type=foundation.enum.transfer_function_type.lag  T=ts s  T1=2 s  T2=1 s  y0=0 m^3/s
      settings: SourceProductBaseCode=SS  InternalSimscapePortConfiguration="{\"Bottom\":[],\"Left\":[{\"id\":\"U\",\"label\":\"\",\"type\":\"input\"}],\"Right\":[{\"id\":\"Y\",\"label\":\"\",\"type\":\"output\"}],\"Top\":[]}"
  PS Transfer Function1 : fl_lib/Physical Signals/Linear Operators/PS Transfer Function  transfer_function_type=foundation.enum.transfer_function_type.lag  T=ts s  T1=2 s  T2=1 s  y0=0 Pa
      settings: SourceProductBaseCode=SS  InternalSimscapePortConfiguration="{\"Bottom\":[],\"Left\":[{\"id\":\"U\",\"label\":\"\",\"type\":\"input\"}],\"Right\":[{\"id\":\"Y\",\"label\":\"\",\"type\":\"output\"}],\"Top\":[]}"
  A : PMIOPort  Side=Left
  B : PMIOPort  Port=2  Side=Right
  connections:
  PS Transfer Function/LConn1 -- PS Saturation/RConn1
  PS Saturation1/RConn1 -- PS Transfer Function1/LConn1
  PS Transfer Function/RConn1 -- Hydraulic Flow Rate Source/RConn1
  Constant Area Hydraulic Orifice5/LConn1 -- A/RConn1 -- Hydraulic Pressure Sensor/LConn1 -- Hydraulic Flow Rate Source/RConn2
  Hydraulic Pressure Sensor/RConn2 -- PS Saturation1/LConn1
  PS Transfer Function1/RConn1 -- Hydraulic Pressure Source2/RConn1
  PS Saturation/LConn1 -- Hydraulic Flow Rate Sensor/RConn1
  B/RConn1 -- Constant Area Hydraulic Orifice5/RConn1 -- Hydraulic Pressure Sensor/RConn1 -- Hydraulic Flow Rate Source/LConn1
  Hydraulic Pressure Source2/LConn1 -- Hydraulic Flow Rate Sensor/LConn1
  Hydraulic Pressure Source2/RConn2 -- Hydraulic Reference/LConn1 -- Constant Area Hydraulic Orifice6/RConn1
  Hydraulic Flow Rate Sensor/RConn2 -- Constant Area Hydraulic Orifice6/LConn1

== matlab function nl_obsv_hydrotrans_dspace/motor_speed_control/EKF/riccati ==
  data: P input; dp_hat input; omega_m_hat input; tau_m_hat input; vp input; vm input; Pdot output; Jp input; Jm input; bp input; bm input; bulk input; Vp_nom input; Vm_nom input; kleak input; kdrag input; bf input; ntg input; L output; q11 input; q22 input; q33 input; q44 input
function [Pdot, L] = riccati(P, dp_hat, omega_m_hat, tau_m_hat, vp, vm, Jp, Jm, bp,...
    bm, bulk, Vp_nom, Vm_nom, kleak, kdrag, bf, ntg, q11, q22, q33, q44)

    a41 = -2/ntg^3*vm*Vm_nom/Jm*kdrag*omega_m_hat;
    a42 = 0;
    a43 = -2/ntg^3*kdrag/(2*Jm)*(2*vm*Vm_nom*dp_hat-tau_m_hat-2*bm*omega_m_hat) + 2/ntg^3*kdrag*bm/Jm*omega_m_hat;
    a44 = 1/ntg^3*kdrag/Jm*omega_m_hat;

    A = [-2*bulk*kleak 2*bulk*vp*Vp_nom -2*bulk*vm*Vm_nom 0; ...
        -vp/Jp*Vp_nom -bp/Jp 0 0; ...
        vm/Jm*Vm_nom 0 -bm/Jm -1/2/Jm; ...
        a41 a42 a43 a44];

    C = [0 1 0 0; 0 0 1 0];

    R = eye(2);
    Q = [q11 0 0 0; 0 q22 0 0; 0 0 q33 0; 0 0 0 q44];

    Pdot = A*P+P*A'+Q-P*C'/(R)*C*P;
    L = P*C'/R;

== matlab function nl_obsv_hydrotrans_dspace/motor_speed_control/EKF/model ==
  data: dp_hat input; omega_p_hat input; omega_m_hat input; tau_m_hat input; tau_p input; vp input; vm input; dp_hat_dot output; omega_p input; omega_m input; L input; Jp input; Jm input; bp input; bm input; bulk input; omega_p_hat_dot output; Vp_nom input; Vm_nom input; omega_m_hat_dot output; tau_m_hat_dot output; kleak input; kdrag input; bf input; ntg input
function [dp_hat_dot, omega_p_hat_dot, omega_m_hat_dot, tau_m_hat_dot] = ...
    dp_obsv(dp_hat, omega_p_hat, omega_m_hat, tau_m_hat, tau_p, vp, vm, ...
    omega_p, omega_m, L, Jp, Jm, bp, bm, bulk, Vp_nom, Vm_nom, kleak, ...
    kdrag, bf, ntg)

    dp_hat_dot = bulk*(2*vp*Vp_nom*omega_p_hat - 2*vm*Vm_nom*omega_m_hat) ...
        -2*kleak*dp_hat + L(1,1)*(omega_p-omega_p_hat) + L(1,2)*(omega_m-omega_m_hat);
    
    omega_p_hat_dot = 1/(2*Jp)*(tau_p - 2*vp*Vp_nom*dp_hat ...
        - 2*bp*omega_p_hat) + L(2,1)*(omega_p-omega_p_hat) + L(2,2)*(omega_m-omega_m_hat);

    omega_m_hat_dot = 1/(2*Jm)*(2*vm*Vm_nom*dp_hat - tau_m_hat ...
        - 2*bm*omega_m_hat) + L(3,1)*(omega_p-omega_p_hat) + L(3,2)*(omega_m-omega_m_hat);
   
    tau_m_hat_dot = -2/ntg^3*kdrag*omega_m_hat/(2*Jm)*(2*vm*Vm_nom*dp_hat-tau_m_hat-2*bm*omega_m_hat) ...
        + L(4,1)*(omega_p-omega_p_hat) + L(4,2)*(omega_m-omega_m_hat);
